simulink model "DRL_Model_PID_Model"  (R2020b)
settings: Solver=VariableStepAuto  StartTime=0.0  StopTime=10  RelTol=1e-3
values from neighbouring files (symbols this model uses):
  A = param{1,1}    [DRL_parameter.m]
  B = param{1,2}    [DRL_parameter.m]
  C = param{1,3}    [DRL_parameter.m]
  cf = 1000    [compare.m]
  D = param{1,4}    [DRL_parameter.m]
  K = param{1,5}    [DRL_parameter.m]
  max_Voltage = 10    [DRL_parameter.m]
libraries: simulink x3, rllib x1
settings Model: Creator=mohammadim  LastModifiedBy=mohammadim

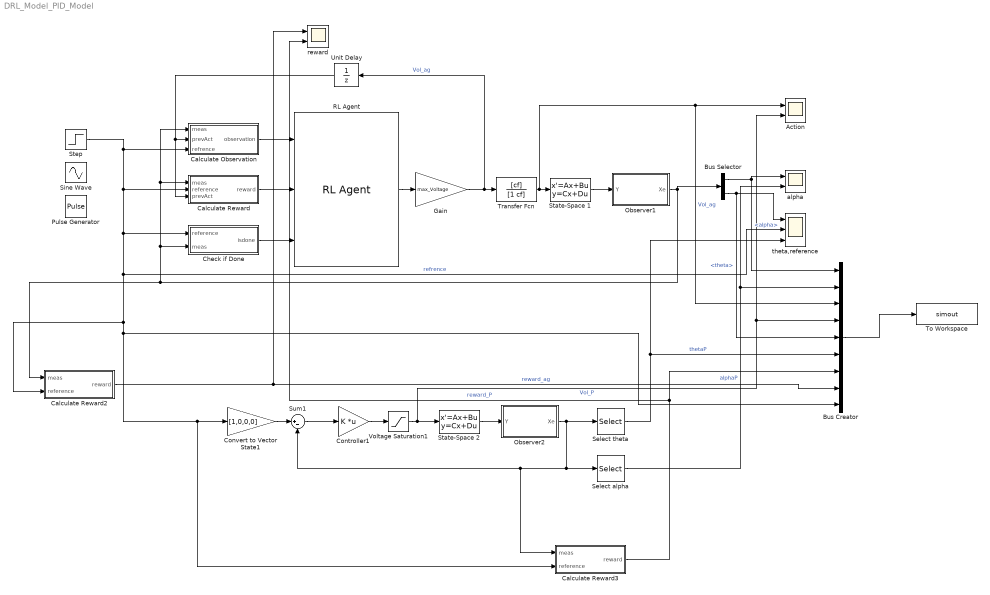
== system DRL_Model_PID_Model ==
  Action : Scope  NumInputPorts=2
  Bus Creator : BusCreator  Inputs=9
  Bus Selector : BusSelector  OutputSignals=alpha,theta
  Calculate Observation : Subsystem
  Calculate Reward : Subsystem
  Calculate Reward2 : Subsystem
  Calculate Reward3 : Subsystem
  Check if Done : Subsystem
  Controller1 : Gain  Gain=K  Multiplication=Matrix(K*u)  SaturateOnIntegerOverflow=on  OutDataTypeStr=Inherit: Same as input  ParamDataTypeStr=Inherit: Same as input
  Convert to Vector State1 : Gain  Gain=[1,0,0,0]
  Gain : Gain  Gain=max_Voltage
  Observer1 : Subsystem
  Observer2 : Subsystem
  Pulse Generator : DiscretePulseGenerator  PulseType=Time based  Period=10  PulseWidth=50
  RL Agent : rllib/RL Agent  Agent=agent  ProvideReward=on  ProvideIsDone=on  ProvideCumRwd=off  TreatAsDirectFeedthrough=on  CollectLoggedSignals=on  CollectModelStates=on
  Select alpha : Selector  InputPortWidth=4  IndexOptions=Index vector (dialog)  Indices=[2]  OutputSizes=1
  Select theta : Selector  InputPortWidth=4  IndexOptions=Index vector (dialog)  Indices=[1]  OutputSizes=1
  Sine Wave : Sin  Frequency=pi  SampleTime=0
  State-Space 1 : StateSpace  A=A  B=B  C=C  D=D  InitialCondition=0
  State-Space 2 : StateSpace  A=A  B=B  C=C  D=D  InitialCondition=0
  Step : Step  SampleTime=0
  Sum1 : Sum  Inputs=|+-
  To Workspace : ToWorkspace  VariableName=simout  SaveFormat=Timeseries  SampleTime=-1
  Transfer Fcn : TransferFcn  Numerator=[cf]  Denominator=[1 cf]
  Unit Delay : UnitDelay  SampleTime=-1  HasFrameUpgradeWarning=on
  Voltage Saturation1 : Saturate  UpperLimit=10  LowerLimit=-10
  alpha : Scope  NumInputPorts=2
  reward : Scope  NumInputPorts=2
  theta,reference : Scope  NumInputPorts=3
  wires:
  Observer1/1(Xe) -> Calculate Reward2/1(meas), Calculate Observation/1(meas), Calculate Reward/1(meas), Check if Done/2(meas), Bus Selector/1
  State-Space 1/1 -> Observer1/1(Y)
  Check if Done/1(isdone) -> RL Agent/3
  Calculate Observation/1(observation) -> RL Agent/1
  Unit Delay/1 -> Calculate Reward/3(prevAct), Calculate Observation/2(prevAct)
  Calculate Reward/1(reward) -> RL Agent/2
  RL Agent/1 -> Gain/1
  Bus Selector/1 -> alpha/1, Bus Creator/1  "<alpha>"
  Bus Selector/2 -> Bus Creator/5, theta,reference/1  "<theta>"
  Step/1 -> Bus Creator/9, Calculate Reward3/2(reference), Convert to Vector State1/1, Calculate Reward2/2(reference), theta,reference/2, Check if Done/1(reference), Calculate Reward/2(reference), Calculate Observation/3(refrence)  "refrence"
  Gain/1 -> Unit Delay/1, Transfer Fcn/1  "Vol_ag"
  Select alpha/1 -> alpha/2, Bus Creator/2  "alphaP"
  Bus Creator/1 -> To Workspace/1
  Select theta/1 -> theta,reference/3, Bus Creator/6  "thetaP"
  Convert to Vector State1/1 -> Sum1/1
  Controller1/1 -> Voltage Saturation1/1
  Voltage Saturation1/1 -> State-Space 2/1, Action/2, Bus Creator/4  "Vol_P"
  State-Space 2/1 -> Observer2/1(Y)
  Observer2/1(Xe) -> Select theta/1, Calculate Reward3/1(meas), Sum1/2, Select alpha/1
  Sum1/1 -> Controller1/1
  Calculate Reward3/1(reward) -> reward/2, Bus Creator/7  "reward_P"
  Calculate Reward2/1(reward) -> reward/1, Bus Creator/8  "reward_ag"
  Transfer Fcn/1 -> Bus Creator/3, Action/1, State-Space 1/1  "Vol_ag"

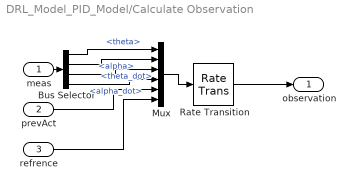
== system DRL_Model_PID_Model/Calculate Observation ==
  meas : Inport
  prevAct : Inport  Port=2
  refrence : Inport  Port=3
  Bus Selector : BusSelector  OutputSignals=theta,alpha,theta_dot,alpha_dot
  Mux : Mux  Inputs=6
  Rate Transition : RateTransition
  observation : Outport  VectorParamsAs1DForOutWhenUnconnected=off
  wires:
  prevAct/1 -> Mux/5
  Rate Transition/1 -> observation/1
  Mux/1 -> Rate Transition/1
  meas/1 -> Bus Selector/1
  Bus Selector/1 -> Mux/1  "<theta>"
  Bus Selector/2 -> Mux/2  "<alpha>"
  Bus Selector/3 -> Mux/3  "<theta_dot>"
  Bus Selector/4 -> Mux/4  "<alpha_dot>"
  refrence/1 -> Mux/6

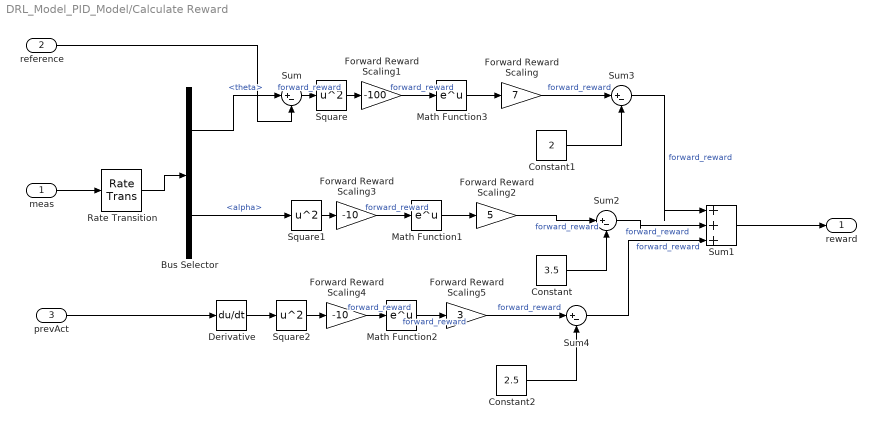
== system DRL_Model_PID_Model/Calculate Reward ==
  meas : Inport
  reference : Inport  Port=2
  prevAct : Inport  Port=3
  Bus Selector : BusSelector  OutputSignals=theta,alpha
  Constant : Constant  Value=3.5
  Constant1 : Constant  Value=2
  Constant2 : Constant  Value=2.5
  Derivative : Derivative
  Forward Reward Scaling : Gain  Gain=7
  Forward Reward Scaling1 : Gain  Gain=-100
  Forward Reward Scaling2 : Gain  Gain=5
  Forward Reward Scaling3 : Gain  Gain=-10
  Forward Reward Scaling4 : Gain  Gain=-10
  Forward Reward Scaling5 : Gain  Gain=3
  Math Function1 : Math  SaturateOnIntegerOverflow=on
  Math Function2 : Math  SaturateOnIntegerOverflow=on
  Math Function3 : Math  SaturateOnIntegerOverflow=on
  Rate Transition : RateTransition  OutPortSampleTime=Ts
  Square : Math  Operator=square  SaturateOnIntegerOverflow=on
  Square1 : Math  Operator=square  SaturateOnIntegerOverflow=on
  Square2 : Math  Operator=square  SaturateOnIntegerOverflow=on
  Sum{,2..4} (4 alike) : Sum  Inputs=|+-
  Sum1 : Sum  Inputs=|+++
  reward : Outport  VectorParamsAs1DForOutWhenUnconnected=off
  wires:
  Rate Transition/1 -> Bus Selector/1
  meas/1 -> Rate Transition/1
  Sum3/1 -> Sum1/1  "forward_reward"
  Sum/1 -> Square/1  "forward_reward"
  Bus Selector/1 -> Sum/1  "<theta>"
  reference/1 -> Sum/2
  Math Function3/1 -> Forward Reward Scaling/1
  Square/1 -> Forward Reward Scaling1/1
  Forward Reward Scaling1/1 -> Math Function3/1  "forward_reward"
  Forward Reward Scaling3/1 -> Math Function1/1  "forward_reward"
  Square1/1 -> Forward Reward Scaling3/1
  Math Function1/1 -> Forward Reward Scaling2/1
  Bus Selector/2 -> Square1/1  "<alpha>"
  Sum1/1 -> reward/1
  Forward Reward Scaling2/1 -> Sum2/1  "forward_reward"
  Constant/1 -> Sum2/2
  Forward Reward Scaling/1 -> Sum3/1  "forward_reward"
  Constant1/1 -> Sum3/2
  prevAct/1 -> Derivative/1
  Derivative/1 -> Square2/1
  Square2/1 -> Forward Reward Scaling4/1
  Sum4/1 -> Sum1/3  "forward_reward"
  Forward Reward Scaling4/1 -> Math Function2/1  "forward_reward"
  Math Function2/1 -> Forward Reward Scaling5/1  "forward_reward"
  Sum2/1 -> Sum1/2  "forward_reward"
  Forward Reward Scaling5/1 -> Sum4/1  "forward_reward"
  Constant2/1 -> Sum4/2

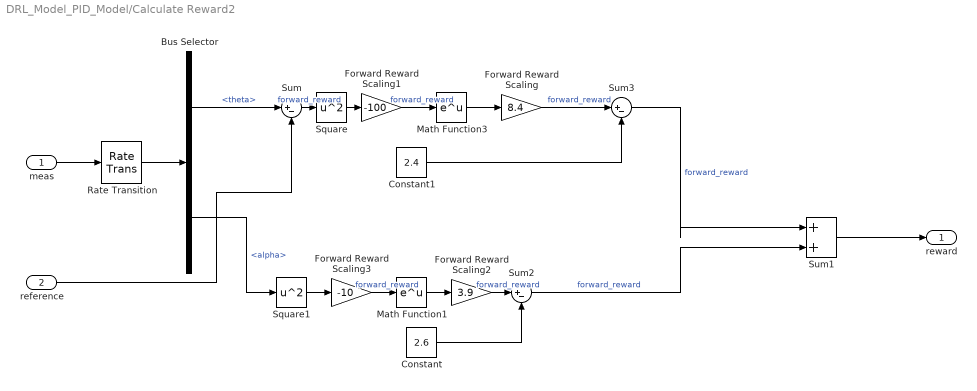
== system DRL_Model_PID_Model/Calculate Reward2 ==
  meas : Inport
  reference : Inport  Port=2
  Bus Selector : BusSelector  OutputSignals=theta,alpha
  Constant : Constant  Value=2.6
  Constant1 : Constant  Value=2.4
  Forward Reward Scaling : Gain  Gain=8.4
  Forward Reward Scaling1 : Gain  Gain=-100
  Forward Reward Scaling2 : Gain  Gain=3.9
  Forward Reward Scaling3 : Gain  Gain=-10
  Math Function1 : Math  SaturateOnIntegerOverflow=on
  Math Function3 : Math  SaturateOnIntegerOverflow=on
  Rate Transition : RateTransition  OutPortSampleTime=Ts
  Square : Math  Operator=square  SaturateOnIntegerOverflow=on
  Square1 : Math  Operator=square  SaturateOnIntegerOverflow=on
  Sum : Sum  Inputs=|+-
  Sum1 : Sum  Inputs=|++
  Sum2 : Sum  Inputs=|+-
  Sum3 : Sum  Inputs=|+-
  reward : Outport  VectorParamsAs1DForOutWhenUnconnected=off
  wires:
  Forward Reward Scaling1/1 -> Math Function3/1  "forward_reward"
  Constant1/1 -> Sum3/2
  Bus Selector/1 -> Sum/1  "<theta>"
  Forward Reward Scaling/1 -> Sum3/1  "forward_reward"
  Square/1 -> Forward Reward Scaling1/1
  meas/1 -> Rate Transition/1
  Math Function3/1 -> Forward Reward Scaling/1
  Sum/1 -> Square/1  "forward_reward"
  Rate Transition/1 -> Bus Selector/1
  reference/1 -> Sum/2
  Math Function1/1 -> Forward Reward Scaling2/1
  Bus Selector/2 -> Square1/1  "<alpha>"
  Forward Reward Scaling3/1 -> Math Function1/1  "forward_reward"
  Forward Reward Scaling2/1 -> Sum2/1  "forward_reward"
  Square1/1 -> Forward Reward Scaling3/1
  Sum2/1 -> Sum1/2  "forward_reward"
  Constant/1 -> Sum2/2
  Sum1/1 -> reward/1
  Sum3/1 -> Sum1/1  "forward_reward"

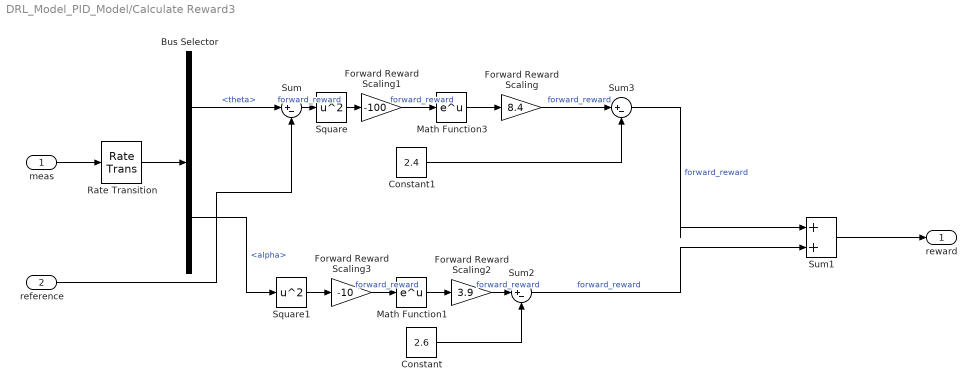
== system DRL_Model_PID_Model/Calculate Reward3 ==
  meas : Inport
  reference : Inport  Port=2
  Bus Selector : BusSelector  OutputSignals=theta,alpha
  Constant : Constant  Value=2.6
  Constant1 : Constant  Value=2.4
  Forward Reward Scaling : Gain  Gain=8.4
  Forward Reward Scaling1 : Gain  Gain=-100
  Forward Reward Scaling2 : Gain  Gain=3.9
  Forward Reward Scaling3 : Gain  Gain=-10
  Math Function1 : Math  SaturateOnIntegerOverflow=on
  Math Function3 : Math  SaturateOnIntegerOverflow=on
  Rate Transition : RateTransition  OutPortSampleTime=Ts
  Square : Math  Operator=square  SaturateOnIntegerOverflow=on
  Square1 : Math  Operator=square  SaturateOnIntegerOverflow=on
  Sum : Sum  Inputs=|+-
  Sum1 : Sum  Inputs=|++
  Sum2 : Sum  Inputs=|+-
  Sum3 : Sum  Inputs=|+-
  reward : Outport  VectorParamsAs1DForOutWhenUnconnected=off
  wires:
  Forward Reward Scaling1/1 -> Math Function3/1  "forward_reward"
  Constant1/1 -> Sum3/2
  Bus Selector/1 -> Sum/1  "<theta>"
  Forward Reward Scaling/1 -> Sum3/1  "forward_reward"
  Square/1 -> Forward Reward Scaling1/1
  meas/1 -> Rate Transition/1
  Math Function3/1 -> Forward Reward Scaling/1
  Sum/1 -> Square/1  "forward_reward"
  Rate Transition/1 -> Bus Selector/1
  reference/1 -> Sum/2
  Math Function1/1 -> Forward Reward Scaling2/1
  Bus Selector/2 -> Square1/1  "<alpha>"
  Forward Reward Scaling3/1 -> Math Function1/1  "forward_reward"
  Forward Reward Scaling2/1 -> Sum2/1  "forward_reward"
  Square1/1 -> Forward Reward Scaling3/1
  Sum2/1 -> Sum1/2  "forward_reward"
  Constant/1 -> Sum2/2
  Sum1/1 -> reward/1
  Sum3/1 -> Sum1/1  "forward_reward"

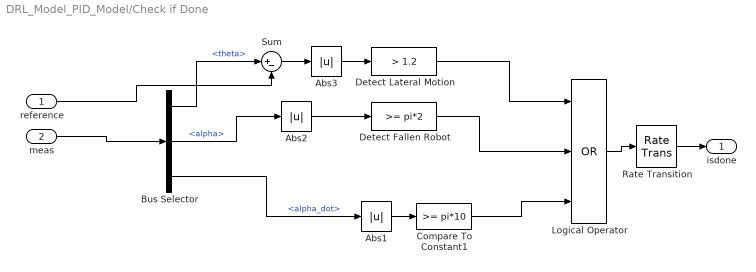
== system DRL_Model_PID_Model/Check if Done ==
  reference : Inport
  meas : Inport  Port=2
  Abs1 : Abs
  Abs2 : Abs
  Abs3 : Abs
  Bus Selector : BusSelector  OutputSignals=theta,alpha,alpha_dot
  Compare To Constant1 : simulink/Logic and Bit Operations/Compare To Constant  relop=>=  const=pi*10  OutDataTypeStr=boolean
  Detect Fallen Robot : simulink/Logic and Bit Operations/Compare To Constant  relop=>=  const=pi*2  OutDataTypeStr=boolean
  Detect Lateral Motion : simulink/Logic and Bit Operations/Compare To Constant  relop=>  const=1.2  OutDataTypeStr=boolean
  Logical Operator : Logic  Operator=OR  Inputs=3  AllPortsSameDT=off  OutDataTypeStr=boolean
  Rate Transition : RateTransition
  Sum : Sum  Inputs=|+-
  isdone : Outport  VectorParamsAs1DForOutWhenUnconnected=off
  wires:
  Detect Lateral Motion/1 -> Logical Operator/1
  Abs3/1 -> Detect Lateral Motion/1
  Rate Transition/1 -> isdone/1
  Compare To Constant1/1 -> Logical Operator/3
  Abs1/1 -> Compare To Constant1/1
  Bus Selector/3 -> Abs1/1  "<alpha_dot>"
  Detect Fallen Robot/1 -> Logical Operator/2
  Logical Operator/1 -> Rate Transition/1
  meas/1 -> Bus Selector/1
  Abs2/1 -> Detect Fallen Robot/1
  Bus Selector/2 -> Abs2/1  "<alpha>"
  Bus Selector/1 -> Sum/1  "<theta>"
  Sum/1 -> Abs3/1
  reference/1 -> Sum/2

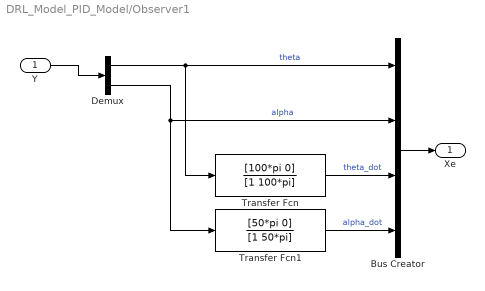
== system DRL_Model_PID_Model/Observer1 ==
  Y : Inport
  Bus Creator : BusCreator  Inputs=4
  Demux : Demux  Outputs=2
  Transfer Fcn : TransferFcn  Numerator=[100*pi 0]  Denominator=[1 100*pi]
  Transfer Fcn1 : TransferFcn  Numerator=[50*pi 0]  Denominator=[1 50*pi]
  Xe : Outport
  wires:
  Transfer Fcn1/1 -> Bus Creator/4  "alpha_dot"
  Demux/1 -> Transfer Fcn/1, Bus Creator/1  "theta"
  Transfer Fcn/1 -> Bus Creator/3  "theta_dot"
  Y/1 -> Demux/1
  Bus Creator/1 -> Xe/1
  Demux/2 -> Transfer Fcn1/1, Bus Creator/2  "alpha"

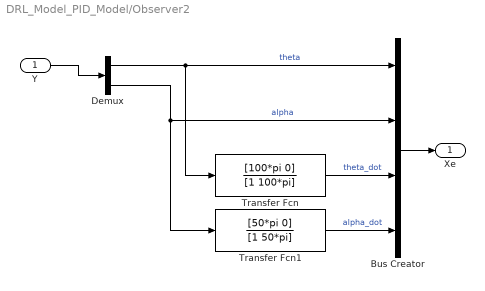
== system DRL_Model_PID_Model/Observer2 ==
  Y : Inport
  Bus Creator : BusCreator  Inputs=4
  Demux : Demux  Outputs=2
  Transfer Fcn : TransferFcn  Numerator=[100*pi 0]  Denominator=[1 100*pi]
  Transfer Fcn1 : TransferFcn  Numerator=[50*pi 0]  Denominator=[1 50*pi]
  Xe : Outport
  wires:
  Demux/2 -> Bus Creator/2, Transfer Fcn1/1  "alpha"
  Bus Creator/1 -> Xe/1
  Y/1 -> Demux/1
  Transfer Fcn/1 -> Bus Creator/3  "theta_dot"
  Demux/1 -> Bus Creator/1, Transfer Fcn/1  "theta"
  Transfer Fcn1/1 -> Bus Creator/4  "alpha_dot"
